simulink model "MPC_cruise_control"  (R2021a)
settings: Solver=VariableStepAuto  StartTime=0.0  StopTime=0.1  RelTol=1e-3
values from neighbouring files (symbols this model uses):
  Cd = 1000    [run_model.m]
  Fr = -Cd*v_star^2    (= -25000)    [run_model.m]
  h = 10    [run_model.m]
  m = 2.7    [run_model.m]
  Q = 2    [run_model.m]
  R = 0.01    [run_model.m]
  Ts = 0.01    [run_model.m]
  v0 = 0    [run_model.m]
  v_star = 5    [run_model.m]
settings Model: Creator=zysgh  LastModifiedBy=zysgh

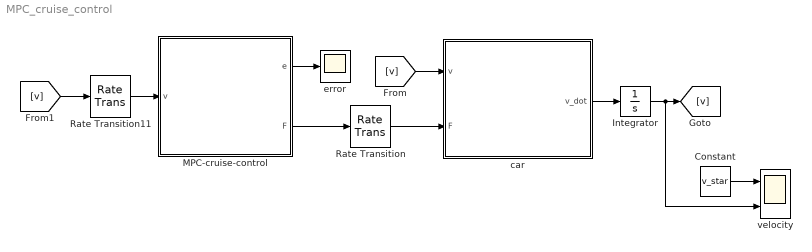
== system MPC_cruise_control ==
  Constant : Constant  Value=v_star
  Integrator : Integrator  InitialCondition=v0
  MPC-cruise-control : MATLAB Function  TreatAsAtomicUnit=on
  Rate Transition : RateTransition  Integrity=off  Deterministic=off  OutPortSampleTime=0
  Rate Transition11 : RateTransition  InitialCondition=v0  OutPortSampleTime=Ts
  car : MATLAB Function  TreatAsAtomicUnit=on
  error : Scope
  velocity : Scope  NumInputPorts=2
  wires:
  car/1(v_dot) -> Integrator/1
  MPC-cruise-control/2(F) -> Rate Transition/1
  Rate Transition/1 -> car/2(F)
  Rate Transition11/1 -> MPC-cruise-control/1(v)
  Integrator/1 -> velocity/2, [v]
  [v] -> car/1(v)
  [v] -> Rate Transition11/1
  MPC-cruise-control/1(e) -> error/1
  Constant/1 -> velocity/1

== matlab function MPC_cruise_control/MPC-cruise-control ==
  data: e output; v input; F output; Cd parameter; Ts parameter; m parameter; Q parameter; R parameter; h parameter; Fr parameter; v_star parameter
function [e,F] = fcn(v,Cd, Ts, m, Q, R, h, Fr, v_star)
%% 

%% error dynamics
A = 1-(2*Cd*Ts*v_star/m);
B = Ts/m;
e = v-v_star;

%% MPC controller
F_fb = optimal_regulation_controller(A,B,-v_star,Q,R,h);

%% control command
F = F_fb * e - Fr;

== matlab function MPC_cruise_control/car ==
  data: v input; v_dot output; F input; m parameter; Cd parameter
function v_dot = fcn(v,F,m, Cd)
%% car longitudinal velocity dynamics, a simplified model
% Inputs:
%        v: longitudinal velocity
%        F: rear wheel force
% Outputs:
%        v_dot: acceleration
%
% Yu Zheng, Raslab, Florida State University, 2022/02/03
%

v_dot = -(Cd/m)*v*v + (1/m)*F;
